simulink model "lab_10"  (R2022b)
settings: Solver=FixedStepAuto  StartTime=0.0  StopTime=10  FixedStep=0.01  RelTol=1e-3
undefined symbols (not defined in the file): A, B, K, K_1, K_2, Q, Q_1, Q_2, R, R_1, R_2
settings Model: Creator=osini  LastModifiedBy=osini

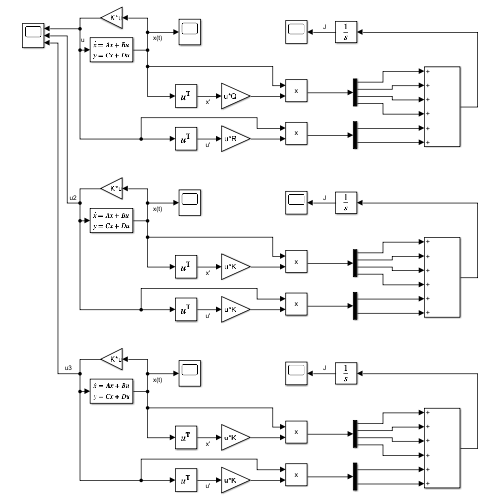
[thumbnail: Simulink's stored preview of the top-level diagram]
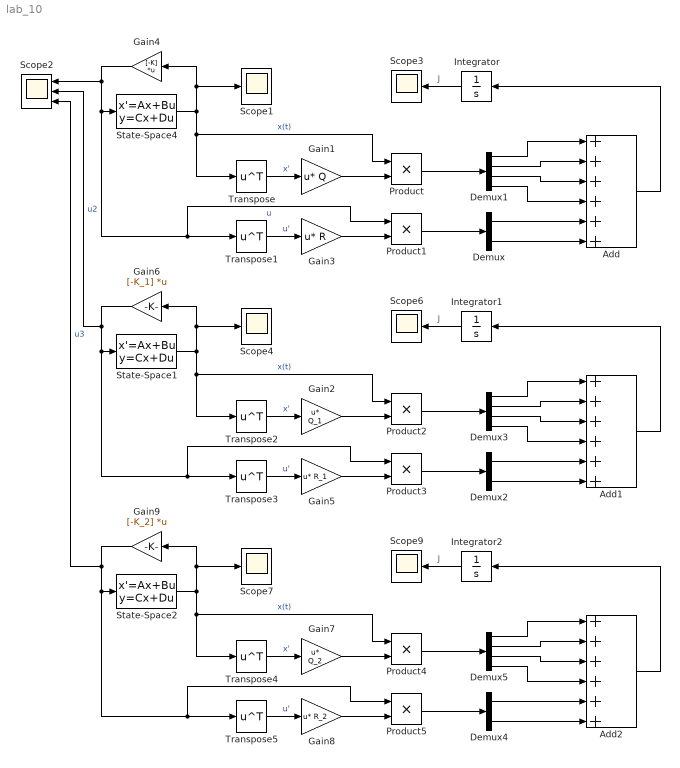
== system lab_10 ==
  Add : Sum  Inputs=++++++
  Add1 : Sum  Inputs=++++++
  Add2 : Sum  Inputs=++++++
  Demux : Demux  Outputs=2
  Demux1 : Demux
  Demux2 : Demux  Outputs=2
  Demux3 : Demux
  Demux4 : Demux  Outputs=2
  Demux5 : Demux
  Gain1 : Gain  Gain=Q  Multiplication=Matrix(u*K)
  Gain2 : Gain  Gain=Q_1  Multiplication=Matrix(u*K)
  Gain3 : Gain  Gain=R  Multiplication=Matrix(u*K)
  Gain4 : Gain  Gain=[-K]  Multiplication=Matrix(K*u)
  Gain5 : Gain  Gain=R_1  Multiplication=Matrix(u*K)
  Gain6 : Gain  Gain=[-K_1]  Multiplication=Matrix(K*u)
  Gain7 : Gain  Gain=Q_2  Multiplication=Matrix(u*K)
  Gain8 : Gain  Gain=R_2  Multiplication=Matrix(u*K)
  Gain9 : Gain  Gain=[-K_2]  Multiplication=Matrix(K*u)
  Integrator : Integrator
  Integrator1 : Integrator
  Integrator2 : Integrator
  Product{,1..5} (6 alike) : Product
  Scope{1,3..4,6..7,9} (6 alike) : Scope
  Scope2 : Scope  NumInputPorts=3
  State-Space1 : StateSpace  A=A  B=B  C=eye(4)  D=zeros(4,2)  InitialCondition=1
  State-Space2 : StateSpace  A=A  B=B  C=eye(4)  D=zeros(4,2)  InitialCondition=1
  State-Space4 : StateSpace  A=A  B=B  C=eye(4)  D=zeros(4,2)  InitialCondition=1
  Transpose{,1..5} (6 alike) : Math  Operator=transpose
  wires:
  Product1/1 -> Demux/1
  Demux1/2 -> Add/2
  Demux/2 -> Add/6
  Demux1/3 -> Add/3
  Demux1/4 -> Add/4
  Demux1/1 -> Add/1
  Transpose/1 -> Gain1/1  "x'"
  Integrator/1 -> Scope3/1  "J"
  Transpose1/1 -> Gain3/1  "u'"
  Gain1/1 -> Product/2
  State-Space4/1 -> Transpose/1, Product/1, Gain4/1, Scope1/1  "x(t)"
  Gain4/1 -> Product1/1, Transpose1/1, State-Space4/1, Scope2/1  "u"
  Gain3/1 -> Product1/2
  Add/1 -> Integrator/1
  Product/1 -> Demux1/1
  Demux/1 -> Add/5
  Add1/1 -> Integrator1/1
  Product2/1 -> Demux3/1
  Demux3/1 -> Add1/1
  Demux2/1 -> Add1/5
  State-Space1/1 -> Transpose2/1, Product2/1, Gain6/1, Scope4/1  "x(t)"
  Integrator1/1 -> Scope6/1  "J"
  Demux3/2 -> Add1/2
  Demux3/4 -> Add1/4
  Gain5/1 -> Product3/2
  Gain2/1 -> Product2/2
  Gain6/1 -> Scope2/2, Product3/1, Transpose3/1, State-Space1/1  "u2"
  Product3/1 -> Demux2/1
  Transpose2/1 -> Gain2/1  "x'"
  Demux2/2 -> Add1/6
  Transpose3/1 -> Gain5/1  "u'"
  Demux3/3 -> Add1/3
  Add2/1 -> Integrator2/1
  Product4/1 -> Demux5/1
  Demux5/1 -> Add2/1
  Demux4/1 -> Add2/5
  State-Space2/1 -> Transpose4/1, Product4/1, Gain9/1, Scope7/1  "x(t)"
  Integrator2/1 -> Scope9/1  "J"
  Demux5/2 -> Add2/2
  Demux5/4 -> Add2/4
  Gain8/1 -> Product5/2
  Gain7/1 -> Product4/2
  Gain9/1 -> Scope2/3, Product5/1, Transpose5/1, State-Space2/1  "u3"
  Product5/1 -> Demux4/1
  Transpose4/1 -> Gain7/1  "x'"
  Demux4/2 -> Add2/6
  Transpose5/1 -> Gain8/1  "u'"
  Demux5/3 -> Add2/3
